simulink model "lab2_1"  (Simulink 7.3)
settings: Solver=ode45  StartTime=1  StopTime=2  RelTol=1e-3
settings Model: Creator=student  LastModifiedBy=student

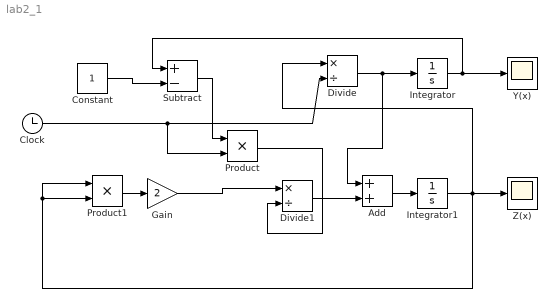
== system lab2_1 ==
  Add : Sum  OutDataType=fixdt(1, 16)  OutScaling=2^-10
  Clock : Clock
      settings: Decimation=10
  Constant : Constant  OutDataType=fixdt(1, 16)  OutScaling=2^0
  Divide : Product  Inputs=*/  OutDataType=fixdt(1, 16)  OutScaling=2^-10
  Divide1 : Product  Inputs=*/  OutDataType=fixdt(1, 16)  OutScaling=2^-10
  Gain : Gain  Gain=2  ParameterDataType=fixdt(1, 16)  ParameterScaling=2^0  OutDataType=fixdt(1, 16)  OutScaling=2^0
  Integrator : Integrator
  Integrator1 : Integrator  InitialCondition=1/3
  Product : Product  OutDataType=fixdt(1, 16)  OutScaling=2^0  RndMeth=Zero
  Product1 : Product  OutDataType=fixdt(1, 16)  OutScaling=2^0  RndMeth=Zero
  Subtract : Sum  Inputs=+-  OutDataType=fixdt(1, 16)  OutScaling=2^-10
  Y(x) : Scope
      settings: Description=11
  Z(x) : Scope
  wires:
  Integrator1/1 -> Divide/1, Product1/1, Product1/2, Z(x)/1
  Clock/1 -> Divide/2, Product/2
  Divide/1 -> Integrator/1, Add/1
  Add/1 -> Integrator1/1
  Product1/1 -> Gain/1
  Integrator/1 -> Subtract/1, Y(x)/1
  Constant/1 -> Subtract/2
  Subtract/1 -> Product/1
  Gain/1 -> Divide1/1
  Product/1 -> Divide1/2
  Divide1/1 -> Add/2
